simulink model "Modelo_Cinematico"  (R2020b)
settings: Solver=VariableStepAuto  StartTime=0.0  StopTime=30  RelTol=1e-3
libraries: simulink x2
settings Model: Creator=danie  LastModifiedBy=danie

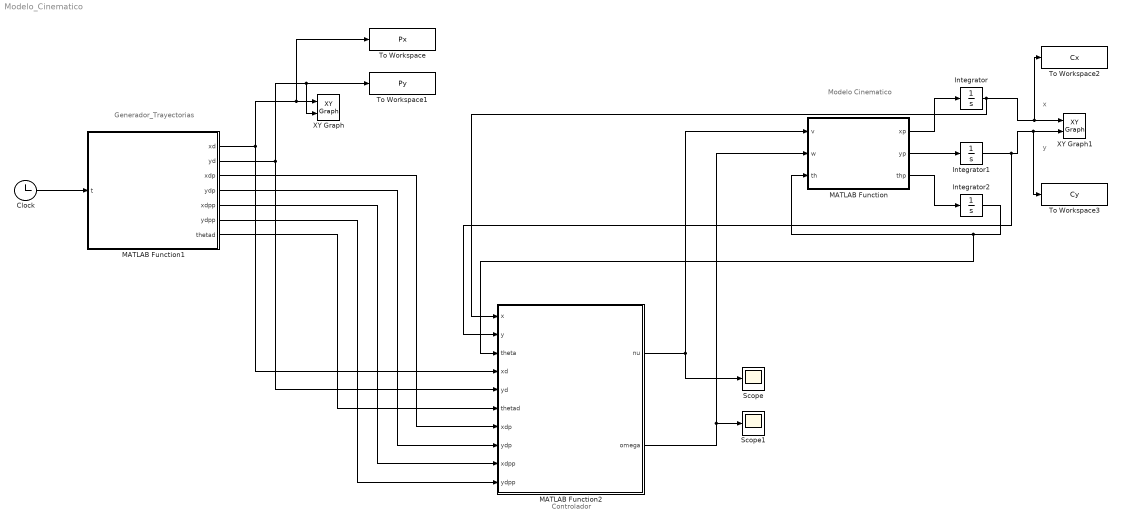
== system Modelo_Cinematico ==
  note: y
  note: x
  note: Controlador
  note: Generador_Trayectorias
  note: Modelo Cinematico
  Clock : Clock
  Integrator : Integrator  InitialCondition=5
  Integrator1 : Integrator
  Integrator2 : Integrator
  MATLAB Function : MATLAB Function  TreatAsAtomicUnit=on
  MATLAB Function1 : MATLAB Function  TreatAsAtomicUnit=on
  MATLAB Function2 : MATLAB Function  TreatAsAtomicUnit=on
  Scope : Scope
  Scope1 : Scope
  To Workspace : ToWorkspace  VariableName=Px  SampleTime=-1
  To Workspace1 : ToWorkspace  VariableName=Py  SampleTime=-1
  To Workspace2 : ToWorkspace  VariableName=Cx  SampleTime=-1
  To Workspace3 : ToWorkspace  VariableName=Cy  SampleTime=-1
  XY Graph : simulink/Sinks/XY Graph  xmin=-10  xmax=10  ymin=-10  ymax=10  st=-1
  XY Graph1 : simulink/Sinks/XY Graph  xmin=-10  xmax=10  ymin=-10  ymax=10  st=-1
  wires:
  MATLAB Function/3(thp) -> Integrator2/1
  Integrator2/1 -> MATLAB Function2/3(theta), MATLAB Function/3(th)
  MATLAB Function/1(xp) -> Integrator/1
  MATLAB Function/2(yp) -> Integrator1/1
  Clock/1 -> MATLAB Function1/1(t)
  MATLAB Function2/1(nu) -> MATLAB Function/1(v), Scope/1
  MATLAB Function2/2(omega) -> MATLAB Function/2(w), Scope1/1
  Integrator/1 -> XY Graph1/1, To Workspace2/1, MATLAB Function2/1(x)
  Integrator1/1 -> MATLAB Function2/2(y), XY Graph1/2, To Workspace3/1
  MATLAB Function1/1(xd) -> XY Graph/1, To Workspace/1, MATLAB Function2/4(xd)
  MATLAB Function1/2(yd) -> XY Graph/2, To Workspace1/1, MATLAB Function2/5(yd)
  MATLAB Function1/3(xdp) -> MATLAB Function2/7(xdp)
  MATLAB Function1/4(ydp) -> MATLAB Function2/8(ydp)
  MATLAB Function1/5(xdpp) -> MATLAB Function2/9(xdpp)
  MATLAB Function1/6(ydpp) -> MATLAB Function2/10(ydpp)
  MATLAB Function1/7(thetad) -> MATLAB Function2/6(thetad)

== matlab function Modelo_Cinematico/MATLAB Function1 ==
  data: xd output; yd output; t input; xdp output; ydp output; xdpp output; ydpp output; thetad output
function [xd, yd, xdp, ydp, xdpp, ydpp, thetad] = fcn(t)

% Ecuacion parametrica de infinito
xd=5*cos(t);
yd=5*sin(2*t);
% Primera derivada ecuación paramétrica
xdp=-5*sin(t);
ydp=10*cos(2*t);
% Segunda derivada ecuación paramétrica
xdpp=-5*cos(t);
ydpp=-20*sin(2*t);

% Ecuacion parametrica de flor rockera
% xd=5+1.5*cos(t)-cos(5*t);
% yd=5+1.5*sin(t)-sin(7*t);
% Primera derivada
% xdp=5*sin(5*t)-1.5*sin(t);
% ydp=1.5*cos(t)-7*cos(7*t);
% Segunda derivada
% xdpp=25*cos(5*t)-1.5*cos(t);
% ydpp=49*sin(7*t)-1.5*sin(t);

thetad=atan2(ydp, xdp)+pi; %orientacion nominal

== matlab function Modelo_Cinematico/MATLAB Function ==
  data: v input; xp output; w input; yp output; thp output; th input
function [xp, yp, thp] = fcn(v, w, th)

xp=v*cos(th);
yp=v*sin(th);
thp=w;

== matlab function Modelo_Cinematico/MATLAB Function2 ==
  data: x input; nu output; omega output; y input; theta input; xd input; yd input; thetad input; xdp input; ydp input; xdpp input; ydpp input
function [nu, omega] = fcn(x, y, theta, xd, yd, thetad, xdp, ydp, xdpp, ydpp)

b=0.5; %grado de libertad adicional
zeta=8; %coeficiente de amortiguamiento

nud=-sqrt(xdp^2+ydp^2); %velocidad lineal deseada
omegad=((ydpp*xdp)-(xdpp*ydp))/(xdp^2+ydp^2); %velocidad angular deseada

k3=2*zeta*sqrt(omegad^2+b*nud^2);
k1=k3;
k2=b*abs(nud);

nu=nud*cos(thetad-theta)+k1*(cos(theta)*(xd-x)+sin(theta)*(yd-y)); %velocidad lineal

omega=omegad+k2*sign(nud)*(cos(theta)*(xd-x)-sin(theta)*(yd-y))+k3*(thetad-theta); %velocidad angular
